simulink model "LQG"  (R2018a)
settings: Solver=VariableStepAuto  StartTime=0.0  StopTime=500  RelTol=1e-3
values from neighbouring files (symbols this model uses):
  A = stateSpaceModel.A    [System_Control.m]    (also in script2.m)
  B = stateSpaceModel.B    [System_Control.m]    (also in script2.m)
  C = stateSpaceModel.C    [System_Control.m]    (also in script2.m)
  Nbar = Nu+K*Nx    [System_Control.m]    (also in script2.m)
  Ts = stateSpaceModel.Ts    [System_Control.m]    (also in script2.m)
undefined symbols (not defined in the file or in its folder): K, M
settings Model: Creator=Gil  LastModifiedBy=Gil
settings DataIOCC: ReturnWorkspaceOutputs=on
settings SFSimCC: SimUseLocalCustomCode=on
settings RTWCC: RTWUseLocalCustomCode=on

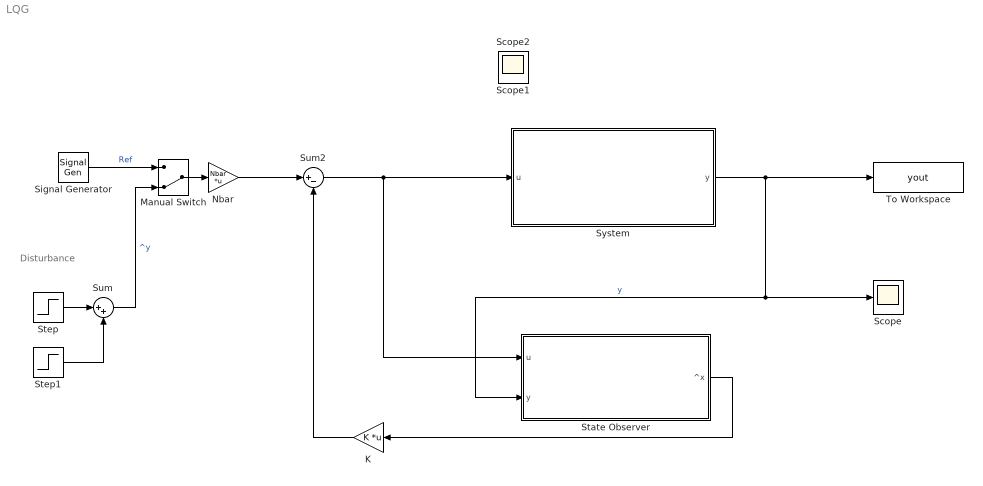
== system LQG ==
  note: Disturbance
  K : Gain  Gain=K  Multiplication=Matrix(K*u)
  Manual Switch : ManualSwitch  CurrentSetting=0
  Nbar : Gain  Gain=Nbar  Multiplication=Matrix(K*u)
  Scope : Scope
  Signal Generator : SignalGenerator  WaveForm=square  Amplitude=5  Frequency=1/50
  State Observer : Subsystem
  Step : Step  Time=2  Before=-1  SampleTime=0.1
  Step1 : Step  Time=4  Before=1  After=-1  SampleTime=0.1
  Sum : Sum  Inputs=|++
  Sum2 : Sum  Inputs=|+-
  System : Subsystem
  To Workspace : ToWorkspace  VariableName=yout  SaveFormat=Structure With Time  SampleTime=Ts
  Scope1 : Scope
  Scope2 : Scope
  wires:
  Step/1 -> Sum/1
  Step1/1 -> Sum/2
  K/1 -> Sum2/2
  State Observer/1(^x) -> K/1
  System/1(y) -> To Workspace/1, State Observer/2(y), Scope/1  "y"
  Sum2/1 -> System/1(u), State Observer/1(u)
  Nbar/1 -> Sum2/1
  Manual Switch/1 -> Nbar/1
  Sum/1 -> Manual Switch/2  "^y"
  Signal Generator/1 -> Manual Switch/1  "Ref"

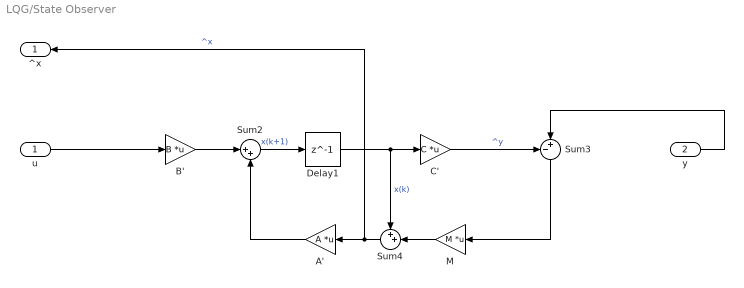
== system LQG/State Observer ==
  u : Inport
  y : Inport  Port=2
  A' : Gain  Gain=A  Multiplication=Matrix(K*u)
  B' : Gain  Gain=B  Multiplication=Matrix(K*u)
  C' : Gain  Gain=C  Multiplication=Matrix(K*u)
  Delay1 : Delay  DelayLength=1  InitialCondition=0  SampleTime=Ts
  M : Gain  Gain=M  Multiplication=Matrix(K*u)
  Sum2 : Sum  Inputs=|++
  Sum3 : Sum  Inputs=-+|
  Sum4 : Sum  Inputs=++|
  ^x : Outport
  wires:
  Sum4/1 -> ^x/1, A'/1  "^x"
  A'/1 -> Sum2/2
  M/1 -> Sum4/2
  B'/1 -> Sum2/1
  Delay1/1 -> Sum4/1, C'/1  "x(k)"
  C'/1 -> Sum3/1  "^y"
  Sum3/1 -> M/1
  y/1 -> Sum3/2
  Sum2/1 -> Delay1/1  "x(k+1)"
  u/1 -> B'/1

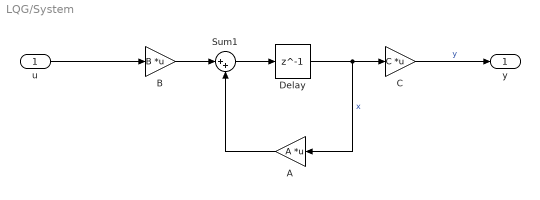
== system LQG/System ==
  u : Inport
  "A " : Gain  Gain=A  Multiplication=Matrix(K*u)
  B : Gain  Gain=B  Multiplication=Matrix(K*u)
  C : Gain  Gain=C  Multiplication=Matrix(K*u)
  Delay : Delay  DelayLength=1  InitialCondition=0  SampleTime=Ts
  Sum1 : Sum  Inputs=|++
  y : Outport
  wires:
  u/1 -> B/1
  "A "/1 -> Sum1/2
  C/1 -> y/1  "y"
  Delay/1 -> "A "/1, C/1  "x"
  Sum1/1 -> Delay/1
  B/1 -> Sum1/1
